simulink model "WEEKEPROB3"  (R2020a)
settings: Solver=VariableStepAuto  StartTime=0.0  StopTime=10.0  RelTol=1e-3
undefined symbols (not defined in the file): DOWN_TABLE, DOWN_TH_BP, UP_TABLE, UP_TH_BP
settings Model: Creator=Admin  LastModifiedBy=Admin

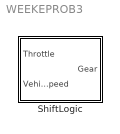
== system WEEKEPROB3 ==
  ShiftLogic : Stateflow chart  TreatAsAtomicUnit=on

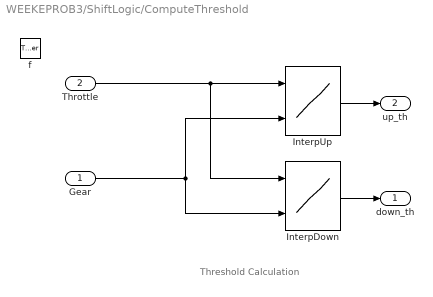
== system WEEKEPROB3/ShiftLogic/ComputeThreshold ==
  note: Threshold Calculation
  Gear : Inport
  Throttle : Inport  Port=2
  f : TriggerPort  TriggerType=function-call  VariantControl=(inherit)
      settings: CopyFcn=Stateflow.SLINSF.SimulinkMan.removeBlockPreDeleteFcn  PreDeleteFcn=Stateflow.SLINSF.SimulinkMan.unsafePredeleteFcn
  InterpDown : Lookup_n-D  BreakpointsForDimension1=DOWN_TH_BP  BreakpointsForDimension2=[1:4]  Table=DOWN_TABLE  OutDataTypeStr=double  LockScale=on
  InterpUp : Lookup_n-D  BreakpointsForDimension1=UP_TH_BP  BreakpointsForDimension2=[1:4]  Table=UP_TABLE  OutDataTypeStr=double  LockScale=on
  down_th : Outport  InitialOutput=0  VectorParamsAs1DForOutWhenUnconnected=off
  up_th : Outport  Port=2  InitialOutput=0  VectorParamsAs1DForOutWhenUnconnected=off
  wires:
  InterpUp/1 -> up_th/1
  InterpDown/1 -> down_th/1
  Throttle/1 -> InterpDown/1, InterpUp/1
  Gear/1 -> InterpDown/2, InterpUp/2

== stateflow chart WEEKEPROB3/ShiftLogic ==
  settings: updateMethod=DISCRETE  sampleTime=0.04
  state gear_state [parallel]
    settings: executionOrder=1
    state first
      entry:
      Gear = 1;
    state second
      entry:
      Gear = 2;
    state third
      entry:
      Gear = 3;
    state fourth
      entry:
      Gear = 4;
    (default) -> first
    second -> third [order 1] : UP
    first -> second : UP
    third -> fourth [order 1] : UP
    third -> second [order 2] : DOWN
    second -> first [order 2] : DOWN
    fourth -> third : DOWN
  state selection_state [parallel]
    during:
    [down_th, up_th] = ComputeThreshold(Gear,Throttle);
    settings: executionOrder=2
    state steady_state
    state upshifting
    state downshifting
    (default) -> steady_state
    steady_state -> upshifting [order 1] : [VehicleSpeed > up_th]
    steady_state -> downshifting [order 2] : [VehicleSpeed < down_th]
    downshifting -> steady_state [order 2] : [VehicleSpeed > down_th]
    downshifting -> steady_state [order 1] : after(TWAIT,tick)
        | [VehicleSpeed <= down_th]
        | {gear_state.DOWN}
    upshifting -> steady_state [order 1] : after(TWAIT,tick)
        | [VehicleSpeed >= up_th]
        | {gear_state.UP}
    upshifting -> steady_state [order 2] : [VehicleSpeed < up_th]
  state [down_th,up_th] = ComputeThreshold(Gear,Throttle) [function]
  data: Gear function_input; Throttle function_input; down_th function_output; up_th function_output; Throttle input double; VehicleSpeed input double; Gear output fixdt(0,8,5) [1..4]; TWAIT parameter fixdt(0,8,6); down_th local double; up_th local double
  events: DOWN local EITHER_EDGE_EVENT; UP local EITHER_EDGE_EVENT
